simulink model "sampleModel1428"  (R2023a)
settings: Solver=VariableStepAuto  StartTime=0.0  StopTime=10.0  RelTol=1e-3
libraries: hdlsllib x6, simulink x1
settings Model: Creator=user1  LastModifiedBy=user1

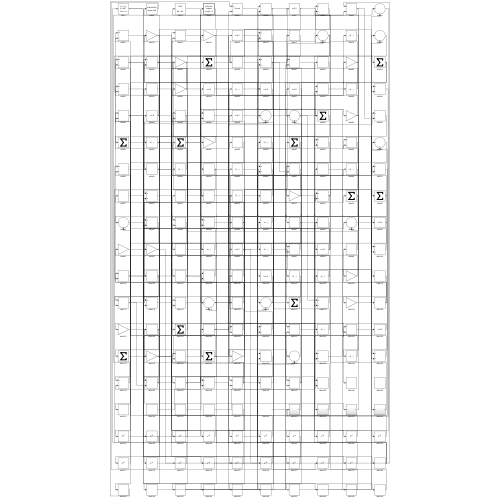
[thumbnail: Simulink's stored preview of the top-level diagram]
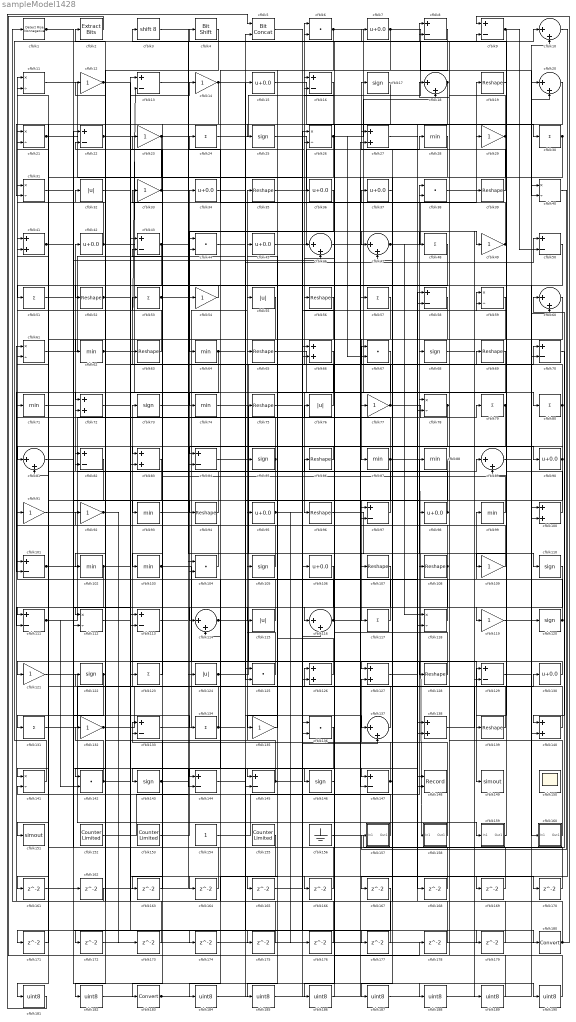
== system sampleModel1428 ==
  cfblk1 : hdlsllib/Logic and Bit Operations/Detect Rise Nonnegative  vinit=0  OutDataTypeStr=boolean
  cfblk{10,18,20,46..47,60,81,89,114,116,137} (11 alike) : Sum  Inputs=|++
  cfblk{27,41,66,72,83,100,126..127,138,140} (10 alike) : Sum
  cfblk{8..9,13,16,22,43,50,58,70,82,84,97,101,111,113,129,133,144..145,147} (20 alike) : Sum  Inputs=+-
  cfblk{28,62,64,71,74,87..88,93,99,102..103} (11 alike) : MinMax
  cfblk{6,38,44,67,104,125,136,142} (8 alike) : DotProduct  OutDataTypeStr=Inherit: Inherit via internal rule
  cfblk{17,25,68,73,85,105,110,120,122,143,146} (11 alike) : Signum
  cfblk{7,15,34,36..37,42,45,90,95,98,106,130} (12 alike) : Bias  Bias=0.0  SaturateOnIntegerOverflow=off
  cfblk{19,35,39,52,56,63,65,69,75,86,94,96,107..108,128,139} (16 alike) : Reshape
  cfblk{12,14,23,29,33,49,54,77,91..92,109,119,121,132,135} (15 alike) : Gain
  cfblk{11,21,26,31,40,59,61,78,112,118,141} (11 alike) : Product  Inputs=*/  RndMeth=Zero  SaturateOnIntegerOverflow=on
  cfblk{32,55,76,115,124} (5 alike) : Abs  SaturateOnIntegerOverflow=off
  cfblk{24,30,48,51,53,57,79..80,117,123,131,134} (12 alike) : Sum  Inputs=+
  cfblk148 : Record  FileSettingsInternal="{\"entries\":[{\"content\":{\"excelSettings\":{\"content\":{},\"type\":\"Streamout.ExcelSettings\"}},\"type\":\"Streamout.FileSettingStorage\",\"uuid\":\"\"}],\"packageUris\":[\"http:\\/\\/schema.mathworks.com\\/mf0\\/streamout_blocks\\/R2020a\"],\"version\":\"1.0\"}"  Layout=[1 1]  SignalsInternal="{\"entries\":[{\"content\":{},\"type\":\"RecordBlkView.InputSignals\",\"uuid\":\"\"}],\"packageUris\":[\"http:\\/\\/schema.mathworks.com\\/mf0\\/streamout_blocks\\/R2020a\"],\"version\":\"1.0\"}"  VisualizationBindings="{\"xyplotplugin\":{\"info\":[{\"series\":[{\"bindingParametersList\":[{\"parameter\":\"X-Axis\",\"signalID\":464,\"signalName\":\"cfblk114\"},{\"parameter\":\"Y-Axis\",\"signalID\":468,\"signalName\":\"cfblk116\"}],\"seriesID\":58657}],\"subplotID\":1}]}}"  CompatibilityTag=XY  st=-1
  cfblk149 : ToWorkspace  VariableName=simout  SaveFormat=Timeseries  SampleTime=-1
  cfblk150 : Scope
      settings: Floating=on
  cfblk151 : ToWorkspace  VariableName=simout  SaveFormat=Timeseries  SampleTime=-1
  cfblk152 : hdlsllib/Sources/Counter Limited  uplimit=7  tsamp=-1
  cfblk153 : hdlsllib/Sources/Counter Limited  uplimit=7  tsamp=-1
  cfblk154 : Constant  SampleTime=-1
  cfblk155 : hdlsllib/Sources/Counter Limited  uplimit=7  tsamp=-1
  cfblk156 : Ground
  cfblk157 : Subsystem
      settings: LibrarySourceBlock=|
      | hdlsllib/Ports &
      | Subsystems/Subsystem
  cfblk158 : Subsystem
      settings: LibrarySourceBlock=|
      | hdlsllib/Ports &
      | Subsystems/Subsystem
  cfblk159 : Subsystem
      settings: LibrarySourceBlock=|
      | hdlsllib/Ports &
      | Subsystems/Subsystem
  cfblk160 : Subsystem
      settings: LibrarySourceBlock=|
      | hdlsllib/Ports &
      | Subsystems/Subsystem
  cfblk{161..179} (19 alike) : Delay  SampleTime=1
  cfblk180 : DataTypeConversion  SaturateOnIntegerOverflow=off  RndMeth=Floor
  cfblk{181..182,184..190} (9 alike) : DataTypeConversion  OutDataTypeStr=uint8  SaturateOnIntegerOverflow=off  RndMeth=Floor
  cfblk183 : DataTypeConversion  SaturateOnIntegerOverflow=off  RndMeth=Floor
  cfblk2 : simulink/Logic and Bit Operations/Extract Bits  bitsToExtract=Upper half  numBits=8  bitIdxRange=[0 7]  outScalingMode=Preserve fixed-point scaling
      settings: LibrarySourceBlock=|
      | hdlsllib/Logic and Bit
      | Operations/Extract Bits
  cfblk3 : ArithShift  BitShiftNumber=8
  cfblk4 : hdlsllib/Logic and Bit Operations/Bit Shift  mode=Shift Left Logical  N=0
  cfblk5 : hdlsllib/Logic and Bit Operations/Bit Concat  numInputs=2
  wires:
  cfblk130/1 -> cfblk121/1
  cfblk76/1 -> cfblk6/1
  cfblk6/1 -> cfblk80/1, cfblk185/1
  cfblk115/1 -> cfblk11/1
  cfblk97/1 -> cfblk42/1
  cfblk153/1 -> cfblk34/1
  cfblk87/1 -> cfblk158/1(In1), cfblk112/2, cfblk61/2
  cfblk131/1 -> cfblk126/1
  cfblk8/1 -> cfblk144/1
  cfblk45/1 -> cfblk49/1
  cfblk91/1 -> cfblk89/1
  cfblk4/1 -> cfblk72/1
  cfblk122/1 -> cfblk32/1, cfblk171/1
  cfblk145/1 -> cfblk35/1, cfblk137/2, cfblk122/1
  cfblk143/1 -> cfblk147/1, cfblk86/1
  cfblk133/1 -> cfblk55/1
  cfblk137/1 -> cfblk73/1
  cfblk66/1 -> cfblk96/1
  cfblk125/1 -> cfblk65/1
  cfblk16/1 -> cfblk103/1
  cfblk154/1 -> cfblk38/1
  cfblk61/1 -> cfblk15/1
  cfblk152/1 -> cfblk124/1
  cfblk5/1 -> cfblk180/1
  cfblk141/1 -> cfblk4/1
  cfblk156/1 -> cfblk60/1
  cfblk79/1 -> cfblk89/2, cfblk115/1
  cfblk36/1 -> cfblk64/1
  cfblk47/1 -> cfblk19/1, cfblk118/1
  cfblk90/1 -> cfblk117/1, cfblk81/1
  cfblk100/1 -> cfblk3/1
  cfblk124/1 -> cfblk70/1, cfblk50/1
  cfblk103/1 -> cfblk149/1, cfblk37/1
  cfblk19/1 -> cfblk139/1
  cfblk39/1 -> cfblk17/1
  cfblk63/1 -> cfblk21/1
  cfblk101/1 -> cfblk78/1, cfblk145/2
  cfblk65/1 -> cfblk87/1
  cfblk118/1 -> cfblk16/1
  cfblk139/1 -> cfblk46/1
  cfblk114/1 -> cfblk148/1, cfblk78/2
  cfblk74/1 -> cfblk110/1
  cfblk129/1 -> cfblk60/2
  cfblk30/1 -> cfblk83/2, cfblk187/1
  cfblk56/1 -> cfblk126/2
  cfblk134/1 -> cfblk101/1, cfblk137/1, cfblk39/1
  cfblk136/1 -> cfblk183/1
  cfblk138/1 -> cfblk130/1
  cfblk120/1 -> cfblk99/1, cfblk23/1
  cfblk42/1 -> cfblk31/1, cfblk140/2
  cfblk102/1 -> cfblk14/1, cfblk111/2
  cfblk60/1 -> cfblk146/1
  cfblk72/1 -> cfblk38/2
  cfblk69/1 -> cfblk135/1
  cfblk135/1 -> cfblk105/1
  cfblk14/1 -> cfblk131/1, cfblk97/2
  cfblk111/1 -> cfblk13/1, cfblk142/2
  cfblk15/1 -> cfblk30/1
  cfblk128/1 -> cfblk92/1
  cfblk17/1 -> cfblk62/1
  cfblk146/1 -> cfblk56/1
  cfblk92/1 -> cfblk172/1, cfblk173/1
  cfblk40/1 -> cfblk157/1(In1)
  cfblk121/1 -> cfblk159/1(In1)
  cfblk24/1 -> cfblk10/1
  cfblk93/1 -> cfblk88/1
  cfblk110/1 -> cfblk114/1
  cfblk31/1 -> cfblk46/2
  cfblk82/1 -> cfblk141/1
  cfblk109/1 -> cfblk45/1
  cfblk41/1 -> cfblk134/1, cfblk174/1
  cfblk106/1 -> cfblk116/1
  cfblk3/1 -> cfblk107/1
  cfblk80/1 -> cfblk22/2, cfblk165/1
  cfblk54/1 -> cfblk52/1
  cfblk11/1 -> cfblk106/1
  cfblk119/1 -> cfblk40/1
  cfblk48/1 -> cfblk102/1
  cfblk132/1 -> cfblk129/1, cfblk69/1, cfblk175/1
  cfblk62/1 -> cfblk13/2, cfblk128/1
  cfblk28/1 -> cfblk147/2
  cfblk22/1 -> cfblk120/1, cfblk142/1, cfblk144/2
  cfblk78/1 -> cfblk18/1, cfblk163/1
  cfblk49/1 -> cfblk24/1, cfblk119/1
  cfblk21/1 -> cfblk125/2, cfblk179/1
  cfblk99/1 -> cfblk53/1
  cfblk35/1 -> cfblk28/1
  cfblk34/1 -> cfblk48/1
  cfblk33/1 -> cfblk90/1, cfblk12/1
  cfblk67/1 -> cfblk145/1
  cfblk9/1 -> cfblk109/1, cfblk50/2
  cfblk46/1 -> cfblk100/1
  cfblk73/1 -> cfblk10/2
  cfblk29/1 -> cfblk44/2, cfblk8/2
  cfblk58/1 -> cfblk77/1
  cfblk57/1 -> cfblk143/1
  cfblk123/1 -> cfblk63/1
  cfblk86/1 -> cfblk84/1
  cfblk12/1 -> cfblk123/1, cfblk112/1
  cfblk52/1 -> cfblk74/1, cfblk166/1
  cfblk108/1 -> cfblk138/2, cfblk43/2, cfblk81/2
  cfblk26/1 -> cfblk84/2, cfblk18/2, cfblk67/2
  cfblk94/1 -> cfblk2/1
  cfblk1/1 -> cfblk113/2, cfblk190/1
  cfblk44/1 -> cfblk85/1
  cfblk98/1 -> cfblk16/2, cfblk8/1, cfblk71/1
  cfblk13/1 -> cfblk47/1
  cfblk85/1 -> cfblk33/1, cfblk182/1
  cfblk160/1(Out1) -> cfblk108/1
  cfblk105/1 -> cfblk95/1
  cfblk107/1 -> cfblk151/1
  cfblk7/1 -> cfblk40/2, cfblk25/1
  cfblk53/1 -> cfblk54/1, cfblk9/2
  cfblk50/1 -> cfblk70/2
  cfblk77/1 -> cfblk79/1, cfblk36/1
  cfblk159/1(Out1) -> cfblk59/1
  cfblk83/1 -> cfblk93/1
  cfblk64/1 -> cfblk127/1, cfblk101/2
  cfblk70/1 -> cfblk140/1
  cfblk37/1 -> cfblk97/1
  cfblk113/1 -> cfblk104/1
  cfblk140/1 -> cfblk91/1
  cfblk116/1 -> cfblk21/2, cfblk148/2
  cfblk84/1 -> cfblk98/1
  cfblk18/1 -> cfblk31/2, cfblk118/2
  cfblk75/1 -> cfblk59/2
  cfblk95/1 -> cfblk67/1, cfblk176/1
  cfblk43/1 -> cfblk51/1, cfblk58/2
  cfblk117/1 -> cfblk41/1
  cfblk157/1(Out1) -> cfblk41/2
  cfblk147/1 -> cfblk127/2, cfblk27/1
  cfblk126/1 -> cfblk75/1
  cfblk96/1 -> cfblk160/1(In1)
  cfblk55/1 -> cfblk83/1
  cfblk71/1 -> cfblk94/1
  cfblk23/1 -> cfblk7/1, cfblk111/1
  cfblk25/1 -> cfblk129/2
  cfblk158/1(Out1) -> cfblk133/1
  cfblk142/1 -> cfblk132/1, cfblk26/2
  cfblk89/1 -> cfblk100/2
  cfblk88/1 -> cfblk114/2
  cfblk38/1 -> cfblk29/1
  cfblk104/1 -> cfblk82/1
  cfblk59/1 -> cfblk161/1
  cfblk161/1 -> cfblk44/1
  cfblk51/1 -> cfblk162/1
  cfblk162/1 -> cfblk1/1
  cfblk163/1 -> cfblk133/2
  cfblk112/1 -> cfblk164/1
  cfblk164/1 -> cfblk113/1
  cfblk165/1 -> cfblk116/2
  cfblk166/1 -> cfblk22/1
  cfblk10/1 -> cfblk167/1
  cfblk127/1 -> cfblk168/1
  cfblk168/1 -> cfblk11/2
  cfblk27/1 -> cfblk169/1
  cfblk169/1 -> cfblk72/2
  cfblk32/1 -> cfblk170/1
  cfblk170/1 -> cfblk58/1
  cfblk171/1 -> cfblk141/2
  cfblk172/1 -> cfblk9/1
  cfblk173/1 -> cfblk43/1
  cfblk174/1 -> cfblk66/2
  cfblk175/1 -> cfblk104/2
  cfblk176/1 -> cfblk61/1
  cfblk144/1 -> cfblk177/1
  cfblk177/1 -> cfblk125/1
  cfblk2/1 -> cfblk178/1
  cfblk178/1 -> cfblk26/1
  cfblk179/1 -> cfblk82/2
  cfblk180/1 -> cfblk47/2, cfblk66/1, cfblk138/1
  cfblk167/1 -> cfblk181/1
  cfblk181/1 -> cfblk5/1
  cfblk182/1 -> cfblk5/2
  cfblk183/1 -> cfblk27/2, cfblk57/1
  cfblk155/1 -> cfblk184/1
  cfblk184/1 -> cfblk136/1
  cfblk185/1 -> cfblk136/2
  cfblk20/1 -> cfblk186/1
  cfblk186/1 -> cfblk76/1
  cfblk187/1 -> cfblk20/1
  cfblk81/1 -> cfblk188/1
  cfblk188/1 -> cfblk20/2
  cfblk68/1 -> cfblk189/1
  cfblk189/1 -> cfblk6/2
  cfblk190/1 -> cfblk68/1

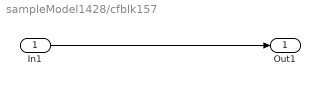
== system sampleModel1428/cfblk157 ==
  In1 : Inport
  Out1 : Outport
  wires:
  In1/1 -> Out1/1

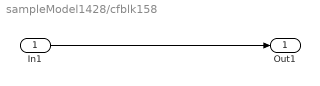
== system sampleModel1428/cfblk158 ==
  In1 : Inport
  Out1 : Outport
  wires:
  In1/1 -> Out1/1

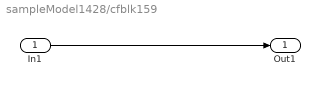
== system sampleModel1428/cfblk159 ==
  In1 : Inport
  Out1 : Outport
  wires:
  In1/1 -> Out1/1

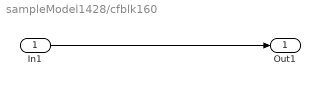
== system sampleModel1428/cfblk160 ==
  In1 : Inport
  Out1 : Outport
  wires:
  In1/1 -> Out1/1
